simulink model "ThreePhaseFullSystemFFT"  (R2021a)
settings: Solver=VariableStepAuto  StartTime=0.0  StopTime=1  RelTol=1e-3
libraries: spsSeriesRLCBranchLib x27, sdolib x6, spsFirstOrderFilterLib x6, dspxfrm3 x3, spsThreePhaseFaultLib x3, spsThreePhaseSeriesRLCLoadLib x1, spsThreePhaseVIMeasurementLib x1, spsThreePhaseSourceLib x1, spspowerguiLib x1, dspsigops x1
settings Model: Creator=ASUS  LastModifiedBy=TUF

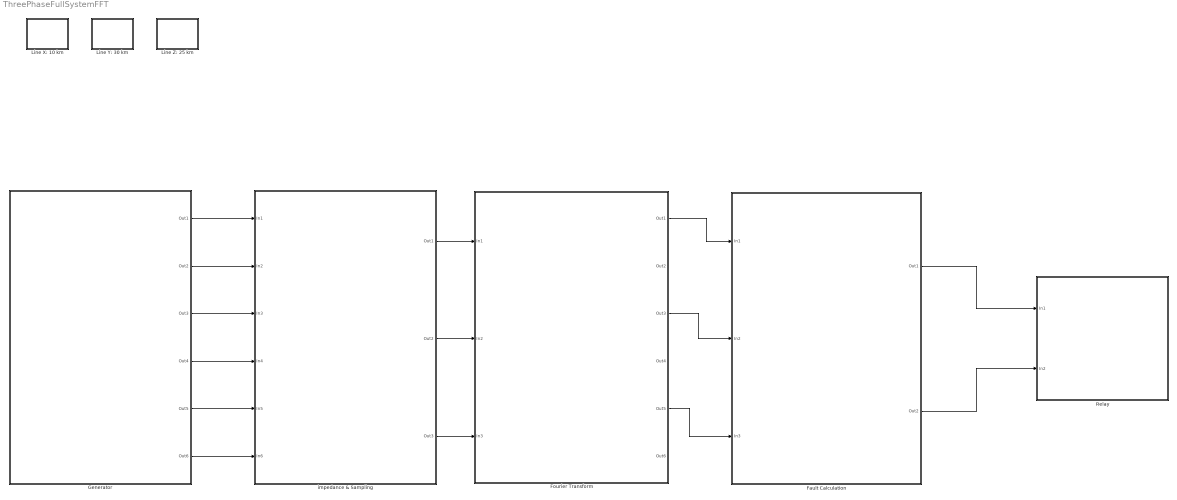
== system ThreePhaseFullSystemFFT ==
  Fault Calculation : Subsystem
  Fourier Transform : Subsystem
  Generator : Subsystem
  Line X: 10 km : Subsystem
  Line Y: 30 km : Subsystem
  Line Z: 25 km : Subsystem
  Relay : Subsystem
  impedance & Sampling : Subsystem
  wires:
  Generator/1(Out1) -> impedance & Sampling/1(In1)
  Generator/2(Out2) -> impedance & Sampling/2(In2)
  Generator/3(Out3) -> impedance & Sampling/3(In3)
  Generator/4(Out4) -> impedance & Sampling/4(In4)
  Generator/5(Out5) -> impedance & Sampling/5(In5)
  Generator/6(Out6) -> impedance & Sampling/6(In6)
  impedance & Sampling/1(Out1) -> Fourier Transform/1(In1)
  impedance & Sampling/2(Out2) -> Fourier Transform/2(In2)
  impedance & Sampling/3(Out3) -> Fourier Transform/3(In3)
  Fourier Transform/1(Out1) -> Fault Calculation/1(In1)
  Fourier Transform/3(Out3) -> Fault Calculation/2(In2)
  Fourier Transform/5(Out5) -> Fault Calculation/3(In3)
  Fault Calculation/1(Out1) -> Relay/1(In1)
  Fault Calculation/2(Out2) -> Relay/2(In2)

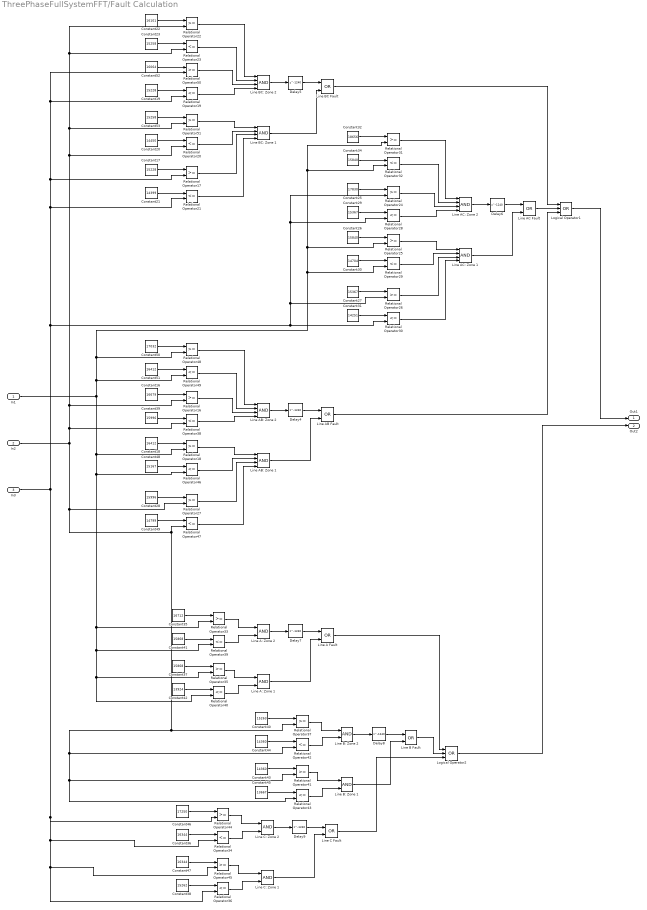
== system ThreePhaseFullSystemFFT/Fault Calculation ==
  In1 : Inport
  In2 : Inport  Port=2
  In3 : Inport  Port=3
  Constant16 : Constant  Value=16679
  Constant17 : Constant  Value=15228
  Constant18 : Constant  Value=16412
  Constant19 : Constant  Value=15228
  Constant20 : Constant  Value=14450
  Constant21 : Constant  Value=14399
  Constant22 : Constant  Value=16101
  Constant23 : Constant  Value=15258
  Constant25 : Constant  Value=17830
  Constant26 : Constant  Value=15840
  Constant27 : Constant  Value=15367
  Constant28 : Constant  Value=15996
  Constant29 : Constant  Value=15367
  Constant30 : Constant  Value=14704
  Constant31 : Constant  Value=14251
  Constant32 : Constant  Value=18656
  Constant34 : Constant  Value=15840
  Constant35 : Constant  Value=16712
  Constant36 : Constant  Value=16344
  Constant37 : Constant  Value=15868
  Constant38 : Constant  Value=15262
  Constant39 : Constant  Value=15996
  Constant40 : Constant  Value=15263
  Constant41 : Constant  Value=15868
  Constant42 : Constant  Value=13924
  Constant43 : Constant  Value=14360
  Constant44 : Constant  Value=14360
  Constant45 : Constant  Value=13667
  Constant46 : Constant  Value=17250
  Constant47 : Constant  Value=16344
  Constant48 : Constant  Value=15167
  Constant49 : Constant  Value=14799
  Constant50 : Constant  Value=17032
  Constant51 : Constant  Value=16412
  Constant52 : Constant  Value=16064
  Constant53 : Constant  Value=15258
  Delay{4..9} (6 alike) : Delay  DelayLength=1240  InitialCondition=0
  Line A Fault : Logic  Operator=OR  AllPortsSameDT=off  OutDataTypeStr=boolean
  Line A: Zone 1 : Logic  AllPortsSameDT=off  OutDataTypeStr=boolean
  Line A: Zone 2 : Logic  AllPortsSameDT=off  OutDataTypeStr=boolean
  Line AB Fault : Logic  Operator=OR  AllPortsSameDT=off  OutDataTypeStr=boolean
  Line AB: Zone 1 : Logic  Inputs=4  AllPortsSameDT=off  OutDataTypeStr=boolean
  Line AB: Zone 2 : Logic  Inputs=4  AllPortsSameDT=off  OutDataTypeStr=boolean
  Line AC Fault : Logic  Operator=OR  AllPortsSameDT=off  OutDataTypeStr=boolean
  Line AC: Zone 1 : Logic  Inputs=4  AllPortsSameDT=off  OutDataTypeStr=boolean
  Line AC: Zone 2 : Logic  Inputs=4  AllPortsSameDT=off  OutDataTypeStr=boolean
  Line B Fault : Logic  Operator=OR  AllPortsSameDT=off  OutDataTypeStr=boolean
  Line B: Zone 1 : Logic  AllPortsSameDT=off  OutDataTypeStr=boolean
  Line B: Zone 2 : Logic  AllPortsSameDT=off  OutDataTypeStr=boolean
  Line BC Fault : Logic  Operator=OR  AllPortsSameDT=off  OutDataTypeStr=boolean
  Line BC: Zone 1 : Logic  Inputs=4  AllPortsSameDT=off  OutDataTypeStr=boolean
  Line BC: Zone 2 : Logic  Inputs=4  AllPortsSameDT=off  OutDataTypeStr=boolean
  Line C Fault : Logic  Operator=OR  AllPortsSameDT=off  OutDataTypeStr=boolean
  Line C: Zone 1 : Logic  AllPortsSameDT=off  OutDataTypeStr=boolean
  Line C: Zone 2 : Logic  AllPortsSameDT=off  OutDataTypeStr=boolean
  Logical Operator1 : Logic  Operator=OR  Inputs=3  AllPortsSameDT=off  OutDataTypeStr=boolean
  Logical Operator2 : Logic  Operator=OR  Inputs=3  AllPortsSameDT=off  OutDataTypeStr=boolean
  Relational Operator{16..18,22,24..27,31,33,35,37,41,44..45,48,50..51} (18 alike) : RelationalOperator  OutDataTypeStr=boolean  RndMeth=Simplest
  Relational Operator{19..21,23,28..30,32,34,36,38..40,42..43,46..47,49} (18 alike) : RelationalOperator  Operator=<=  OutDataTypeStr=boolean  RndMeth=Simplest
  Out1 : Outport
  Out2 : Outport  Port=2
  wires:
  Relational Operator46/1 -> Line AB: Zone 1/2
  Relational Operator17/1 -> Line BC: Zone 1/3
  In2/1 -> Relational Operator27/2, Relational Operator47/2, Relational Operator43/2, Relational Operator41/2, Relational Operator42/2, Relational Operator37/2, Relational Operator20/2, Relational Operator51/2, Relational Operator23/2, Relational Operator22/2, Relational Operator16/2, Relational Operator38/2
  Relational Operator39/1 -> Line A: Zone 2/2
  Constant20/1 -> Relational Operator20/1
  Line C: Zone 2/1 -> Delay9/1
  In1/1 -> Relational Operator29/2, Relational Operator25/2, Relational Operator32/2, Relational Operator31/2, Relational Operator48/2, Relational Operator49/2, Relational Operator18/2, Relational Operator46/2, Relational Operator40/2, Relational Operator35/2, Relational Operator39/2, Relational Operator33/2
  Relational Operator25/1 -> Line AC: Zone 1/1
  Line B Fault/1 -> Logical Operator2/2
  Constant21/1 -> Relational Operator21/1
  Relational Operator18/1 -> Line AB: Zone 1/1
  Constant29/1 -> Relational Operator28/1
  Constant47/1 -> Relational Operator45/1
  Line AC: Zone 1/1 -> Line AC Fault/2
  Line A Fault/1 -> Logical Operator2/1
  Constant26/1 -> Relational Operator25/1
  Line AC: Zone 2/1 -> Delay6/1
  Constant17/1 -> Relational Operator17/1
  Delay9/1 -> Line C Fault/1
  In3/1 -> Relational Operator36/2, Relational Operator45/2, Relational Operator34/2, Relational Operator44/2, Relational Operator21/2, Relational Operator17/2, Relational Operator19/2, Relational Operator50/2, Relational Operator30/2, Relational Operator24/2, Relational Operator28/2, Relational Operator26/2
  Line A: Zone 2/1 -> Delay7/1
  Constant50/1 -> Relational Operator48/1
  Relational Operator47/1 -> Line AB: Zone 1/4
  Relational Operator36/1 -> Line C: Zone 1/2
  Line C Fault/1 -> Logical Operator2/3
  Constant39/1 -> Relational Operator38/1
  Constant43/1 -> Relational Operator41/1
  Delay7/1 -> Line A Fault/1
  Constant23/1 -> Relational Operator23/1
  Relational Operator22/1 -> Line BC: Zone 2/1
  Constant41/1 -> Relational Operator39/1
  Constant52/1 -> Relational Operator50/1
  Constant25/1 -> Relational Operator24/1
  Constant28/1 -> Relational Operator27/1
  Line BC Fault/1 -> Logical Operator1/1
  Relational Operator29/1 -> Line AC: Zone 1/2
  Relational Operator48/1 -> Line AB: Zone 2/1
  Relational Operator44/1 -> Line C: Zone 2/1
  Constant35/1 -> Relational Operator33/1
  Relational Operator19/1 -> Line BC: Zone 2/4
  Relational Operator24/1 -> Line AC: Zone 2/3
  Line BC: Zone 1/1 -> Line BC Fault/2
  Relational Operator30/1 -> Line AC: Zone 1/4
  Relational Operator41/1 -> Line B: Zone 1/1
  Line A: Zone 1/1 -> Line A Fault/2
  Constant37/1 -> Relational Operator35/1
  Line B: Zone 2/1 -> Delay8/1
  Relational Operator50/1 -> Line BC: Zone 2/3
  Constant16/1 -> Relational Operator16/1
  Relational Operator45/1 -> Line C: Zone 1/1
  Relational Operator42/1 -> Line B: Zone 2/2
  Constant36/1 -> Relational Operator34/1
  Delay6/1 -> Line AC Fault/1
  Relational Operator43/1 -> Line B: Zone 1/2
  Constant42/1 -> Relational Operator40/1
  Line BC: Zone 2/1 -> Delay5/1
  Relational Operator35/1 -> Line A: Zone 1/1
  Constant18/1 -> Relational Operator18/1
  Constant46/1 -> Relational Operator44/1
  Relational Operator23/1 -> Line BC: Zone 2/2
  Constant22/1 -> Relational Operator22/1
  Constant49/1 -> Relational Operator47/1
  Relational Operator28/1 -> Line AC: Zone 2/4
  Constant45/1 -> Relational Operator43/1
  Relational Operator20/1 -> Line BC: Zone 1/2
  Relational Operator38/1 -> Line AB: Zone 2/4
  Relational Operator33/1 -> Line A: Zone 2/1
  Constant27/1 -> Relational Operator26/1
  Constant53/1 -> Relational Operator51/1
  Relational Operator40/1 -> Line A: Zone 1/2
  Constant31/1 -> Relational Operator30/1
  Constant40/1 -> Relational Operator37/1
  Relational Operator37/1 -> Line B: Zone 2/1
  Line AB: Zone 1/1 -> Line AB Fault/2
  Relational Operator16/1 -> Line AB: Zone 2/3
  Line AB: Zone 2/1 -> Delay4/1
  Relational Operator26/1 -> Line AC: Zone 1/3
  Line AB Fault/1 -> Logical Operator1/3
  Relational Operator51/1 -> Line BC: Zone 1/1
  Constant32/1 -> Relational Operator31/1
  Relational Operator27/1 -> Line AB: Zone 1/3
  Line C: Zone 1/1 -> Line C Fault/2
  Relational Operator34/1 -> Line C: Zone 2/2
  Line B: Zone 1/1 -> Line B Fault/2
  Delay4/1 -> Line AB Fault/1
  Line AC Fault/1 -> Logical Operator1/2
  Relational Operator49/1 -> Line AB: Zone 2/2
  Constant34/1 -> Relational Operator32/1
  Delay5/1 -> Line BC Fault/1
  Delay8/1 -> Line B Fault/1
  Constant38/1 -> Relational Operator36/1
  Constant48/1 -> Relational Operator46/1
  Constant44/1 -> Relational Operator42/1
  Constant30/1 -> Relational Operator29/1
  Relational Operator31/1 -> Line AC: Zone 2/1
  Relational Operator32/1 -> Line AC: Zone 2/2
  Constant51/1 -> Relational Operator49/1
  Relational Operator21/1 -> Line BC: Zone 1/4
  Constant19/1 -> Relational Operator19/1
  Logical Operator2/1 -> Out2/1
  Logical Operator1/1 -> Out1/1

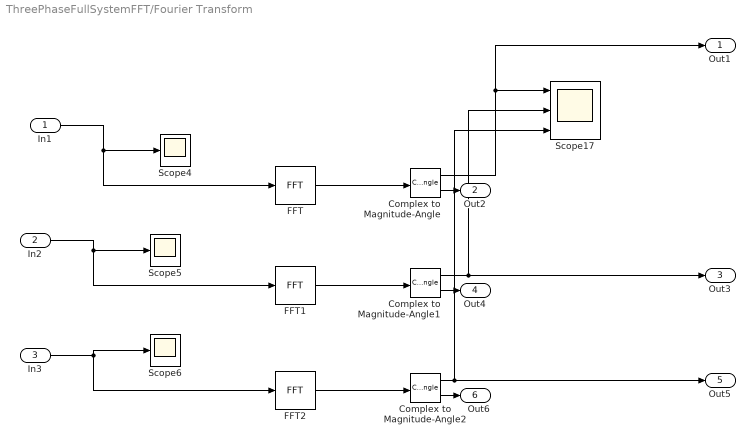
== system ThreePhaseFullSystemFFT/Fourier Transform ==
  In1 : Inport
  In2 : Inport  Port=2
  In3 : Inport  Port=3
  Complex to Magnitude-Angle : ComplexToMagnitudeAngle
  Complex to Magnitude-Angle1 : ComplexToMagnitudeAngle
  Complex to Magnitude-Angle2 : ComplexToMagnitudeAngle
  FFT : dspxfrm3/FFT  FFTImplementation=Auto  CompMethod=Table lookup  TableOpt=NEW  TableOptActive=Speed  BitRevOrder=off  Normalize=off  InheritFFTLength=on  FFTLength=64  WrapInput=on  roundingMode=Floor  overflowMode=off  firstCoeffDataTypeStr=Inherit: Same word length as input  firstCoeffLastDataTypeStr=Inherit: Same word length as input  outputMin=[]  outputMax=[]
  FFT1 : dspxfrm3/FFT  FFTImplementation=Auto  CompMethod=Table lookup  TableOpt=NEW  TableOptActive=Speed  BitRevOrder=off  Normalize=off  InheritFFTLength=on  FFTLength=64  WrapInput=on  roundingMode=Floor  overflowMode=off  firstCoeffDataTypeStr=Inherit: Same word length as input  firstCoeffLastDataTypeStr=Inherit: Same word length as input  outputMin=[]  outputMax=[]
  FFT2 : dspxfrm3/FFT  FFTImplementation=Auto  CompMethod=Table lookup  TableOpt=NEW  TableOptActive=Speed  BitRevOrder=off  Normalize=off  InheritFFTLength=on  FFTLength=64  WrapInput=on  roundingMode=Floor  overflowMode=off  firstCoeffDataTypeStr=Inherit: Same word length as input  firstCoeffLastDataTypeStr=Inherit: Same word length as input  outputMin=[]  outputMax=[]
  Scope17 : Scope  NumInputPorts=3
  Scope4 : Scope
  Scope5 : Scope
  Scope6 : Scope
  Out1 : Outport
  Out2 : Outport  Port=2
  Out3 : Outport  Port=3
  Out4 : Outport  Port=4
  Out5 : Outport  Port=5
  Out6 : Outport  Port=6
  wires:
  In1/1 -> FFT/1, Scope4/1
  FFT2/1 -> Complex to Magnitude-Angle2/1
  Complex to Magnitude-Angle/1 -> Out1/1, Scope17/1
  In3/1 -> Scope6/1, FFT2/1
  Complex to Magnitude-Angle1/1 -> Out3/1, Scope17/2
  In2/1 -> FFT1/1, Scope5/1
  Complex to Magnitude-Angle2/1 -> Out5/1, Scope17/3
  FFT/1 -> Complex to Magnitude-Angle/1
  FFT1/1 -> Complex to Magnitude-Angle1/1
  Complex to Magnitude-Angle/2 -> Out2/1
  Complex to Magnitude-Angle2/2 -> Out6/1
  Complex to Magnitude-Angle1/2 -> Out4/1

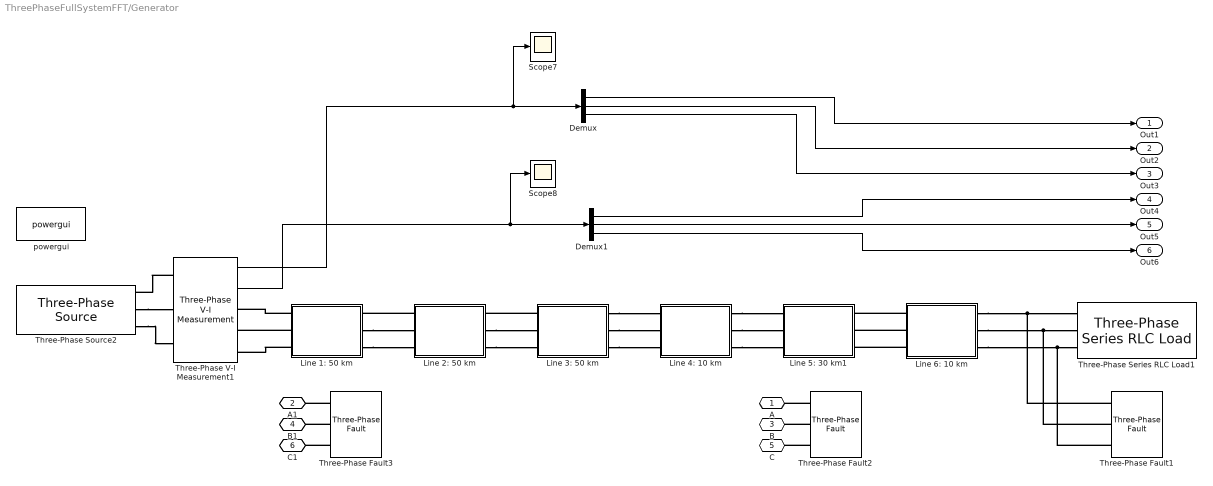
== system ThreePhaseFullSystemFFT/Generator ==
  Demux : Demux  Outputs=3
  Demux1 : Demux  Outputs=3
  Line 1: 50 km : Subsystem
  Line 2: 50 km : Subsystem
  Line 3: 50 km : Subsystem
  Line 4: 10 km : Subsystem
  Line 5: 30 km1 : Subsystem
  Line 6: 10 km : Subsystem
  Scope7 : Scope
  Scope8 : Scope
  Three-Phase Series RLC Load1 : spsThreePhaseSeriesRLCLoadLib/Three-Phase Series RLC Load  LConnTagsString=A|B|C  Configuration=Y (grounded)  NominalVoltage=132e3  Vabc=[1e3 1e3 1e3]  Vabcp=[1e3 1e3 1e3]  NominalFrequency=60  UnbalancedPower=off  ActivePower=600e3  InductivePower=0  CapacitivePower=0  Pabc=[10e3 9e3 11e3]  QLabc=[100 90 110]  QCabc=[100 90 110]  Pabcp=[10e3 9e3 11e3]  QLabcp=[100 90 110]  QCabcp=[100 90 110]  Measurements=None  LoadType=constant Z
  Three-Phase V-I Measurement1 : spsThreePhaseVIMeasurementLib/Three-Phase V-I Measurement  VoltageMeasurement=phase-to-ground  SetLabelV=off  LabelV=Vabc  Vpu=off  VpuLL=off  CurrentMeasurement=yes  SetLabelI=off  LabelI=Iabc  Ipu=off  Pbase=100e6  Vbase=500e3  OutputType=Complex  PhasorSimulation=off  PSBequivalent=0
  Three-Phase Fault1 : spsThreePhaseFaultLib/Three-Phase Fault  InitialStates=0  FaultA=off  FaultB=on  FaultC=on  GroundFault=off  SwitchTimes=[0.5 3]  External=off  SwitchStatus=NaN  FaultResistance=5  GroundResistance=0.05  SnubberResistance=inf  SnubberCapacitance=0  Measurements=None
  Three-Phase Fault2 : spsThreePhaseFaultLib/Three-Phase Fault  InitialStates=0  FaultA=off  FaultB=on  FaultC=on  GroundFault=off  SwitchTimes=[0.5 3]  External=off  SwitchStatus=NaN  FaultResistance=5  GroundResistance=0.05  SnubberResistance=inf  SnubberCapacitance=0  Measurements=None
  Three-Phase Fault3 : spsThreePhaseFaultLib/Three-Phase Fault  InitialStates=0  FaultA=off  FaultB=on  FaultC=on  GroundFault=off  SwitchTimes=[0.5 3]  External=off  SwitchStatus=NaN  FaultResistance=5  GroundResistance=0.05  SnubberResistance=inf  SnubberCapacitance=0  Measurements=None
  Three-Phase Source2 : spsThreePhaseSourceLib/Three-Phase Source  InternalConnection=Yg  VoltagePhases=off  Voltage=132e3  PhaseAngle=0  Voltage_phases=[25e3 25e3 25e3]/sqrt(3)  PhaseAngles_phases=[0 -120 +120]  Frequency=60  NonIdealSource=on  SpecifyImpedance=on  Resistance=0.01134  Inductance=10  ShortCircuitLevel=200e6  BaseVoltage=132e3  XRratio=100  BusType=swing  Pref=180e6  Qref=0  Prefabc=[10e3, 10e3, 10e3]  Qrefabc=[0, 0, 0]  Qmin=-inf  Qmax=inf
  powergui : spspowerguiLib/powergui  Priority=1  SimulationMode=Continuous  SampleTime=3e-05  frequency=60  Iterations=50  frequencyindice=60  Pbase=100e6  ErrMax=1e-4  UnitsV=kV  UnitsW=MW  buscounter=0  FunctionMessages=off  echomessages=off  EnableUseOfTLC=off  CurrentSourceSwitches=off  DisableSnubberDevices=off  DisableRonSwitches=off  DisableVfSwitches=off  DisplayEquations=off  AutomaticDiscreteSolvers=off  SolverType=Tustin/Backward Euler (TBE)  Interpol=off  ExternalGateDelay=off  methode=off  Ts=100  x0status=steady  SPID=on  SwTol=0  HookPort=off  NonlinearTolerance=1e-4  nMaxIteration=100  ContinueOnMaxIteration=off  RestoreLinks=warning  ResistiveCurrentMeasurement=off  Frange=[0:2:500]  Ylog=off  Xlog=on  ShowGrid=off  save=off  variable=ZData  structure=0  ZoomFFT=off  StartTime=0.0  cycles=1  DisplayStyle=1  fundamental=60  FreqAxis=off  MaxFrequency=1000  frequencyindicesteady=1  RmsSteady=1  display=off
  A : PMIOPort  Side=Left
  A1 : PMIOPort  Port=2  Side=Left
  B : PMIOPort  Port=3  Side=Left
  B1 : PMIOPort  Port=4  Side=Left
  C : PMIOPort  Port=5  Side=Left
  C1 : PMIOPort  Port=6  Side=Left
  Out1 : Outport
  Out2 : Outport  Port=2
  Out3 : Outport  Port=3
  Out4 : Outport  Port=4
  Out5 : Outport  Port=5
  Out6 : Outport  Port=6
  wires:
  Demux/3 -> Out3/1
  Three-Phase V-I Measurement1/1 -> Demux/1, Scope7/1
  Three-Phase V-I Measurement1/2 -> Demux1/1, Scope8/1
  Demux1/3 -> Out6/1
  Demux1/1 -> Out4/1
  Demux/1 -> Out1/1
  Demux1/2 -> Out5/1
  Demux/2 -> Out2/1
  connections:
  Three-Phase Fault3/LConn1 -- A1/RConn1
  Three-Phase Fault2/LConn3 -- C/RConn1
  Line 2: 50 km/RConn2 -- Line 3: 50 km/LConn2
  Line 2: 50 km/LConn1 -- Line 1: 50 km/RConn1
  Line 3: 50 km/RConn1 -- Line 4: 10 km/LConn1
  Line 3: 50 km/RConn2 -- Line 4: 10 km/LConn2
  Line 4: 10 km/RConn2 -- Line 5: 30 km1/LConn2
  Line 6: 10 km/LConn1 -- Line 5: 30 km1/RConn1
  Line 1: 50 km/LConn3 -- Three-Phase V-I Measurement1/RConn3
  Line 1: 50 km/RConn3 -- Line 2: 50 km/LConn3
  Line 3: 50 km/RConn3 -- Line 4: 10 km/LConn3
  Line 6: 10 km/RConn3 -- Three-Phase Fault1/LConn3 -- Three-Phase Series RLC Load1/LConn3
  Line 1: 50 km/LConn2 -- Three-Phase V-I Measurement1/RConn2
  Three-Phase Fault2/LConn1 -- A/RConn1
  Line 6: 10 km/RConn2 -- Three-Phase Fault1/LConn2 -- Three-Phase Series RLC Load1/LConn2
  Line 6: 10 km/RConn1 -- Three-Phase Fault1/LConn1 -- Three-Phase Series RLC Load1/LConn1
  Three-Phase Fault2/LConn2 -- B/RConn1
  Three-Phase Fault3/LConn3 -- C1/RConn1
  Three-Phase V-I Measurement1/LConn1 -- Three-Phase Source2/RConn1
  Line 6: 10 km/LConn2 -- Line 5: 30 km1/RConn2
  Line 1: 50 km/LConn1 -- Three-Phase V-I Measurement1/RConn1
  Line 1: 50 km/RConn2 -- Line 2: 50 km/LConn2
  Line 3: 50 km/LConn1 -- Line 2: 50 km/RConn1
  Three-Phase Source2/RConn3 -- Three-Phase V-I Measurement1/LConn3
  Three-Phase Fault3/LConn2 -- B1/RConn1
  Line 4: 10 km/RConn1 -- Line 5: 30 km1/LConn1
  Line 2: 50 km/RConn3 -- Line 3: 50 km/LConn3
  Line 4: 10 km/RConn3 -- Line 5: 30 km1/LConn3
  Line 6: 10 km/LConn3 -- Line 5: 30 km1/RConn3
  Three-Phase Source2/RConn2 -- Three-Phase V-I Measurement1/LConn2

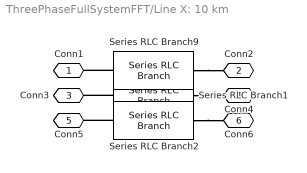
== system ThreePhaseFullSystemFFT/Line X: 10 km ==
  Series RLC Branch1 : spsSeriesRLCBranchLib/Series RLC Branch  LConnTagsString=__new0  RConnTagsString=__new0  BranchType=RL  Resistance=1.134  Inductance=0.83e-2  SetiL0=off  InitialCurrent=0  Capacitance=5.12e-7  Setx0=off  InitialVoltage=0  Measurements=None
  Series RLC Branch2 : spsSeriesRLCBranchLib/Series RLC Branch  LConnTagsString=__new0  RConnTagsString=__new0  BranchType=RL  Resistance=1.134  Inductance=0.83e-2  SetiL0=off  InitialCurrent=0  Capacitance=5.12e-7  Setx0=off  InitialVoltage=0  Measurements=None
  Series RLC Branch9 : spsSeriesRLCBranchLib/Series RLC Branch  LConnTagsString=__new0  RConnTagsString=__new0  BranchType=RL  Resistance=1.134  Inductance=0.83e-2  SetiL0=off  InitialCurrent=0  Capacitance=5.12e-7  Setx0=off  InitialVoltage=0  Measurements=None
  Conn1 : PMIOPort  Side=Left
  Conn2 : PMIOPort  Port=2  Side=Right
  Conn3 : PMIOPort  Port=3  Side=Left
  Conn4 : PMIOPort  Port=4  Side=Right
  Conn5 : PMIOPort  Port=5  Side=Left
  Conn6 : PMIOPort  Port=6  Side=Right
  connections:
  Series RLC Branch9/LConn1 -- Conn1/RConn1
  Series RLC Branch2/LConn1 -- Conn5/RConn1
  Series RLC Branch1/LConn1 -- Conn3/RConn1
  Series RLC Branch2/RConn1 -- Conn6/RConn1
  Series RLC Branch9/RConn1 -- Conn2/RConn1
  Series RLC Branch1/RConn1 -- Conn4/RConn1

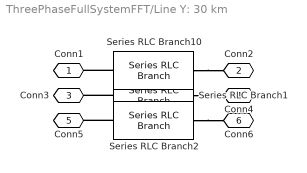
== system ThreePhaseFullSystemFFT/Line Y: 30 km ==
  Series RLC Branch1 : spsSeriesRLCBranchLib/Series RLC Branch  LConnTagsString=__new0  RConnTagsString=__new0  BranchType=RL  Resistance=3.402  Inductance=2.49e-2  SetiL0=off  InitialCurrent=0  Capacitance=5.12e-7  Setx0=off  InitialVoltage=0  Measurements=None
  Series RLC Branch10 : spsSeriesRLCBranchLib/Series RLC Branch  LConnTagsString=__new0  RConnTagsString=__new0  BranchType=RL  Resistance=3.402  Inductance=2.49e-2  SetiL0=off  InitialCurrent=0  Capacitance=5.12e-7  Setx0=off  InitialVoltage=0  Measurements=None
  Series RLC Branch2 : spsSeriesRLCBranchLib/Series RLC Branch  LConnTagsString=__new0  RConnTagsString=__new0  BranchType=RL  Resistance=3.402  Inductance=2.49e-2  SetiL0=off  InitialCurrent=0  Capacitance=5.12e-7  Setx0=off  InitialVoltage=0  Measurements=None
  Conn1 : PMIOPort  Side=Left
  Conn2 : PMIOPort  Port=2  Side=Right
  Conn3 : PMIOPort  Port=3  Side=Left
  Conn4 : PMIOPort  Port=4  Side=Right
  Conn5 : PMIOPort  Port=5  Side=Left
  Conn6 : PMIOPort  Port=6  Side=Right
  connections:
  Series RLC Branch10/LConn1 -- Conn1/RConn1
  Series RLC Branch1/LConn1 -- Conn3/RConn1
  Series RLC Branch1/RConn1 -- Conn4/RConn1
  Series RLC Branch10/RConn1 -- Conn2/RConn1
  Series RLC Branch2/LConn1 -- Conn5/RConn1
  Series RLC Branch2/RConn1 -- Conn6/RConn1

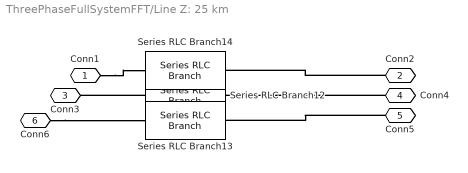
== system ThreePhaseFullSystemFFT/Line Z: 25 km ==
  Series RLC Branch12 : spsSeriesRLCBranchLib/Series RLC Branch  LConnTagsString=__new0  RConnTagsString=__new0  BranchType=RL  Resistance=2.835  Inductance=2.075e-2  SetiL0=off  InitialCurrent=0  Capacitance=5.12e-7  Setx0=off  InitialVoltage=0  Measurements=None
  Series RLC Branch13 : spsSeriesRLCBranchLib/Series RLC Branch  LConnTagsString=__new0  RConnTagsString=__new0  BranchType=RL  Resistance=2.835  Inductance=2.075e-2  SetiL0=off  InitialCurrent=0  Capacitance=5.12e-7  Setx0=off  InitialVoltage=0  Measurements=None
  Series RLC Branch14 : spsSeriesRLCBranchLib/Series RLC Branch  LConnTagsString=__new0  RConnTagsString=__new0  BranchType=RL  Resistance=2.835  Inductance=2.075e-2  SetiL0=off  InitialCurrent=0  Capacitance=5.12e-7  Setx0=off  InitialVoltage=0  Measurements=None
  Conn1 : PMIOPort  Side=Left
  Conn2 : PMIOPort  Port=2  Side=Right
  Conn3 : PMIOPort  Port=3  Side=Left
  Conn4 : PMIOPort  Port=4  Side=Right
  Conn5 : PMIOPort  Port=5  Side=Right
  Conn6 : PMIOPort  Port=6  Side=Left
  connections:
  Conn6/RConn1 -- Series RLC Branch13/LConn1
  Series RLC Branch12/LConn1 -- Conn3/RConn1
  Conn4/RConn1 -- Series RLC Branch12/RConn1
  Conn2/RConn1 -- Series RLC Branch14/RConn1
  Conn5/RConn1 -- Series RLC Branch13/RConn1
  Conn1/RConn1 -- Series RLC Branch14/LConn1

== system ThreePhaseFullSystemFFT/Relay ==
  In1 : Inport
  In2 : Inport  Port=2
  Constant33 : Constant
  Line A Fault3 : Logic  Operator=OR  AllPortsSameDT=off  OutDataTypeStr=boolean
  Relay1 : Scope
  Sample and Hold1 : dspsigops/Sample and Hold  trig=Rising edge  initCond=0  latchinput=off
  wires:
  Line A Fault3/1 -> Sample and Hold1/Trigger
  Constant33/1 -> Sample and Hold1/1
  Sample and Hold1/1 -> Relay1/1
  In1/1 -> Line A Fault3/1
  In2/1 -> Line A Fault3/2

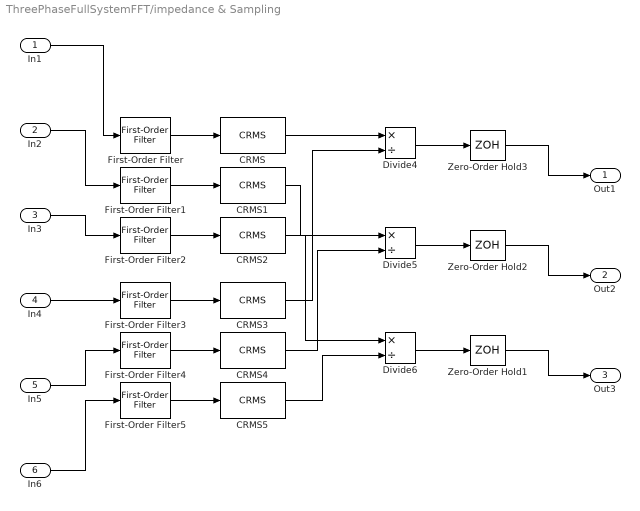
== system ThreePhaseFullSystemFFT/impedance & Sampling ==
  In1 : Inport
  In2 : Inport  Port=2
  In3 : Inport  Port=3
  In4 : Inport  Port=4
  In5 : Inport  Port=5
  In6 : Inport  Port=6
  CRMS{,1..5} (6 alike) : sdolib/RMS Blocks/CRMS
      settings: SourceProductBaseCode=SO
  Divide4 : Product  Inputs=*/
  Divide5 : Product  Inputs=*/
  Divide6 : Product  Inputs=*/
  First-Order Filter{,1..5} (6 alike) : spsFirstOrderFilterLib/First-Order Filter  FilterType=Lowpass  Tc=14e-4  Ts=0  Initialize=on  Vac_Init=[0, 0, 60]  Vdc_Init=0  PlotResponse=off  FreqRange="[0,  200,  1]"
  Zero-Order Hold1 : ZeroOrderHold  SampleTime=0.00025
  Zero-Order Hold2 : ZeroOrderHold  SampleTime=0.00025
  Zero-Order Hold3 : ZeroOrderHold  SampleTime=0.00025
  Out1 : Outport
  Out2 : Outport  Port=2
  Out3 : Outport  Port=3
  wires:
  In4/1 -> First-Order Filter3/1
  First-Order Filter4/1 -> CRMS4/1
  First-Order Filter/1 -> CRMS/1
  First-Order Filter3/1 -> CRMS3/1
  Divide6/1 -> Zero-Order Hold1/1
  CRMS/1 -> Divide4/1
  In3/1 -> First-Order Filter2/1
  CRMS4/1 -> Divide5/2
  CRMS1/1 -> Divide5/1
  CRMS2/1 -> Divide6/1
  CRMS5/1 -> Divide6/2
  First-Order Filter1/1 -> CRMS1/1
  First-Order Filter2/1 -> CRMS2/1
  Divide5/1 -> Zero-Order Hold2/1
  First-Order Filter5/1 -> CRMS5/1
  Divide4/1 -> Zero-Order Hold3/1
  CRMS3/1 -> Divide4/2
  In6/1 -> First-Order Filter5/1
  Zero-Order Hold2/1 -> Out2/1
  Zero-Order Hold1/1 -> Out3/1
  Zero-Order Hold3/1 -> Out1/1
  In1/1 -> First-Order Filter/1
  In5/1 -> First-Order Filter4/1
  In2/1 -> First-Order Filter1/1

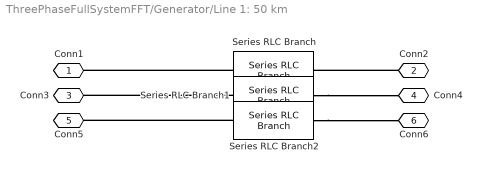
== system ThreePhaseFullSystemFFT/Generator/Line 1: 50 km ==
  Series RLC Branch : spsSeriesRLCBranchLib/Series RLC Branch  LConnTagsString=__new0  RConnTagsString=__new0  BranchType=RL  Resistance=5.67  Inductance=4.15e-2  SetiL0=off  InitialCurrent=0  Capacitance=1.025e-6  Setx0=off  InitialVoltage=0  Measurements=None
  Series RLC Branch1 : spsSeriesRLCBranchLib/Series RLC Branch  LConnTagsString=__new0  RConnTagsString=__new0  BranchType=RL  Resistance=5.67  Inductance=4.15e-2  SetiL0=off  InitialCurrent=0  Capacitance=0  Setx0=off  InitialVoltage=0  Measurements=None
  Series RLC Branch2 : spsSeriesRLCBranchLib/Series RLC Branch  LConnTagsString=__new0  RConnTagsString=__new0  BranchType=RL  Resistance=5.67  Inductance=4.15e-2  SetiL0=off  InitialCurrent=0  Capacitance=1.025e-6  Setx0=off  InitialVoltage=0  Measurements=None
  Conn1 : PMIOPort  Side=Left
  Conn2 : PMIOPort  Port=2  Side=Right
  Conn3 : PMIOPort  Port=3  Side=Left
  Conn4 : PMIOPort  Port=4  Side=Right
  Conn5 : PMIOPort  Port=5  Side=Left
  Conn6 : PMIOPort  Port=6  Side=Right
  connections:
  Series RLC Branch2/RConn1 -- Conn6/RConn1
  Series RLC Branch2/LConn1 -- Conn5/RConn1
  Series RLC Branch1/LConn1 -- Conn3/RConn1
  Conn2/RConn1 -- Series RLC Branch/RConn1
  Series RLC Branch1/RConn1 -- Conn4/RConn1
  Series RLC Branch/LConn1 -- Conn1/RConn1

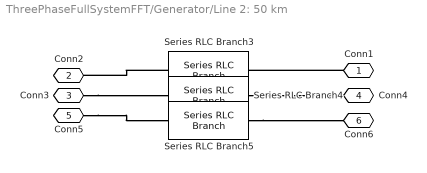
== system ThreePhaseFullSystemFFT/Generator/Line 2: 50 km ==
  Series RLC Branch3 : spsSeriesRLCBranchLib/Series RLC Branch  LConnTagsString=__new0  RConnTagsString=__new0  BranchType=RL  Resistance=5.67  Inductance=4.15e-2  SetiL0=off  InitialCurrent=0  Capacitance=1.025e-6  Setx0=off  InitialVoltage=0  Measurements=None
  Series RLC Branch4 : spsSeriesRLCBranchLib/Series RLC Branch  LConnTagsString=__new0  RConnTagsString=__new0  BranchType=RL  Resistance=5.67  Inductance=4.15e-2  SetiL0=off  InitialCurrent=0  Capacitance=1.025e-6  Setx0=off  InitialVoltage=0  Measurements=None
  Series RLC Branch5 : spsSeriesRLCBranchLib/Series RLC Branch  LConnTagsString=__new0  RConnTagsString=__new0  BranchType=RL  Resistance=5.67  Inductance=4.15e-2  SetiL0=off  InitialCurrent=0  Capacitance=1.025e-6  Setx0=off  InitialVoltage=0  Measurements=None
  Conn1 : PMIOPort  Side=Right
  Conn2 : PMIOPort  Port=2  Side=Left
  Conn3 : PMIOPort  Port=3  Side=Left
  Conn4 : PMIOPort  Port=4  Side=Right
  Conn5 : PMIOPort  Port=5  Side=Left
  Conn6 : PMIOPort  Port=6  Side=Right
  connections:
  Series RLC Branch3/LConn1 -- Conn2/RConn1
  Series RLC Branch5/RConn1 -- Conn6/RConn1
  Series RLC Branch4/RConn1 -- Conn4/RConn1
  Conn3/RConn1 -- Series RLC Branch4/LConn1
  Conn1/RConn1 -- Series RLC Branch3/RConn1
  Conn5/RConn1 -- Series RLC Branch5/LConn1

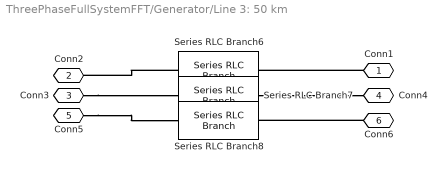
== system ThreePhaseFullSystemFFT/Generator/Line 3: 50 km ==
  Series RLC Branch6 : spsSeriesRLCBranchLib/Series RLC Branch  LConnTagsString=__new0  RConnTagsString=__new0  BranchType=RL  Resistance=5.67  Inductance=4.15e-2  SetiL0=off  InitialCurrent=0  Capacitance=1.025e-6  Setx0=off  InitialVoltage=0  Measurements=None
  Series RLC Branch7 : spsSeriesRLCBranchLib/Series RLC Branch  LConnTagsString=__new0  RConnTagsString=__new0  BranchType=RL  Resistance=5.67  Inductance=4.15e-2  SetiL0=off  InitialCurrent=0  Capacitance=1.025e-6  Setx0=off  InitialVoltage=0  Measurements=None
  Series RLC Branch8 : spsSeriesRLCBranchLib/Series RLC Branch  LConnTagsString=__new0  RConnTagsString=__new0  BranchType=RL  Resistance=5.67  Inductance=4.15e-2  SetiL0=off  InitialCurrent=0  Capacitance=1.025e-6  Setx0=off  InitialVoltage=0  Measurements=None
  Conn1 : PMIOPort  Side=Right
  Conn2 : PMIOPort  Port=2  Side=Left
  Conn3 : PMIOPort  Port=3  Side=Left
  Conn4 : PMIOPort  Port=4  Side=Right
  Conn5 : PMIOPort  Port=5  Side=Left
  Conn6 : PMIOPort  Port=6  Side=Right
  connections:
  Conn6/RConn1 -- Series RLC Branch8/RConn1
  Conn1/RConn1 -- Series RLC Branch6/RConn1
  Conn3/RConn1 -- Series RLC Branch7/LConn1
  Series RLC Branch7/RConn1 -- Conn4/RConn1
  Series RLC Branch6/LConn1 -- Conn2/RConn1
  Conn5/RConn1 -- Series RLC Branch8/LConn1

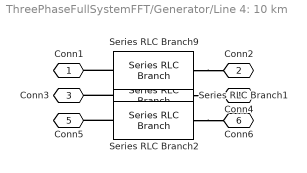
== system ThreePhaseFullSystemFFT/Generator/Line 4: 10 km ==
  Series RLC Branch1 : spsSeriesRLCBranchLib/Series RLC Branch  LConnTagsString=__new0  RConnTagsString=__new0  BranchType=RL  Resistance=1.134  Inductance=0.83e-2  SetiL0=off  InitialCurrent=0  Capacitance=5.12e-7  Setx0=off  InitialVoltage=0  Measurements=None
  Series RLC Branch2 : spsSeriesRLCBranchLib/Series RLC Branch  LConnTagsString=__new0  RConnTagsString=__new0  BranchType=RL  Resistance=1.134  Inductance=0.83e-2  SetiL0=off  InitialCurrent=0  Capacitance=5.12e-7  Setx0=off  InitialVoltage=0  Measurements=None
  Series RLC Branch9 : spsSeriesRLCBranchLib/Series RLC Branch  LConnTagsString=__new0  RConnTagsString=__new0  BranchType=RL  Resistance=1.134  Inductance=0.83e-2  SetiL0=off  InitialCurrent=0  Capacitance=5.12e-7  Setx0=off  InitialVoltage=0  Measurements=None
  Conn1 : PMIOPort  Side=Left
  Conn2 : PMIOPort  Port=2  Side=Right
  Conn3 : PMIOPort  Port=3  Side=Left
  Conn4 : PMIOPort  Port=4  Side=Right
  Conn5 : PMIOPort  Port=5  Side=Left
  Conn6 : PMIOPort  Port=6  Side=Right
  connections:
  Series RLC Branch9/LConn1 -- Conn1/RConn1
  Series RLC Branch2/LConn1 -- Conn5/RConn1
  Series RLC Branch1/LConn1 -- Conn3/RConn1
  Series RLC Branch2/RConn1 -- Conn6/RConn1
  Series RLC Branch9/RConn1 -- Conn2/RConn1
  Series RLC Branch1/RConn1 -- Conn4/RConn1

== system ThreePhaseFullSystemFFT/Generator/Line 5: 30 km1 ==
  Series RLC Branch1 : spsSeriesRLCBranchLib/Series RLC Branch  LConnTagsString=__new0  RConnTagsString=__new0  BranchType=RL  Resistance=3.402  Inductance=2.49e-2  SetiL0=off  InitialCurrent=0  Capacitance=5.12e-7  Setx0=off  InitialVoltage=0  Measurements=None
  Series RLC Branch10 : spsSeriesRLCBranchLib/Series RLC Branch  LConnTagsString=__new0  RConnTagsString=__new0  BranchType=RL  Resistance=3.402  Inductance=2.49e-2  SetiL0=off  InitialCurrent=0  Capacitance=5.12e-7  Setx0=off  InitialVoltage=0  Measurements=None
  Series RLC Branch2 : spsSeriesRLCBranchLib/Series RLC Branch  LConnTagsString=__new0  RConnTagsString=__new0  BranchType=RL  Resistance=3.402  Inductance=2.49e-2  SetiL0=off  InitialCurrent=0  Capacitance=5.12e-7  Setx0=off  InitialVoltage=0  Measurements=None
  Conn1 : PMIOPort  Side=Left
  Conn2 : PMIOPort  Port=2  Side=Right
  Conn3 : PMIOPort  Port=3  Side=Left
  Conn4 : PMIOPort  Port=4  Side=Right
  Conn5 : PMIOPort  Port=5  Side=Left
  Conn6 : PMIOPort  Port=6  Side=Right
  connections:
  Series RLC Branch10/LConn1 -- Conn1/RConn1
  Series RLC Branch1/LConn1 -- Conn3/RConn1
  Series RLC Branch1/RConn1 -- Conn4/RConn1
  Series RLC Branch10/RConn1 -- Conn2/RConn1
  Series RLC Branch2/LConn1 -- Conn5/RConn1
  Series RLC Branch2/RConn1 -- Conn6/RConn1

== system ThreePhaseFullSystemFFT/Generator/Line 6: 10 km ==
  Series RLC Branch1 : spsSeriesRLCBranchLib/Series RLC Branch  LConnTagsString=__new0  RConnTagsString=__new0  BranchType=RL  Resistance=1.134  Inductance=0.83e-2  SetiL0=off  InitialCurrent=0  Capacitance=5.12e-7  Setx0=off  InitialVoltage=0  Measurements=None
  Series RLC Branch2 : spsSeriesRLCBranchLib/Series RLC Branch  LConnTagsString=__new0  RConnTagsString=__new0  BranchType=RL  Resistance=1.134  Inductance=0.83e-2  SetiL0=off  InitialCurrent=0  Capacitance=5.12e-7  Setx0=off  InitialVoltage=0  Measurements=None
  Series RLC Branch9 : spsSeriesRLCBranchLib/Series RLC Branch  LConnTagsString=__new0  RConnTagsString=__new0  BranchType=RL  Resistance=1.134  Inductance=0.83e-2  SetiL0=off  InitialCurrent=0  Capacitance=5.12e-7  Setx0=off  InitialVoltage=0  Measurements=None
  Conn1 : PMIOPort  Side=Left
  Conn3 : PMIOPort  Port=2  Side=Left
  Conn5 : PMIOPort  Port=3  Side=Left
  Conn4 : PMIOPort  Port=4  Side=Right
  Conn2 : PMIOPort  Port=5  Side=Right
  Conn6 : PMIOPort  Port=6  Side=Right
  connections:
  Series RLC Branch9/LConn1 -- Conn1/RConn1
  Series RLC Branch2/LConn1 -- Conn5/RConn1
  Series RLC Branch1/LConn1 -- Conn3/RConn1
  Series RLC Branch2/RConn1 -- Conn6/RConn1
  Series RLC Branch9/RConn1 -- Conn2/RConn1
  Series RLC Branch1/RConn1 -- Conn4/RConn1
